simulink model "w1p2"  (R2020b)
settings: Solver=VariableStepAuto  StartTime=0.0  StopTime=100  MaxStep=0.0001  RelTol=1e-3
model workspace (MAT data in the model file):
  b = 20
  k1 = 50
  k2 = 200
  m1 = 150
  m2 = 100
settings Model: Creator=Puru Gawande  LastModifiedBy=family

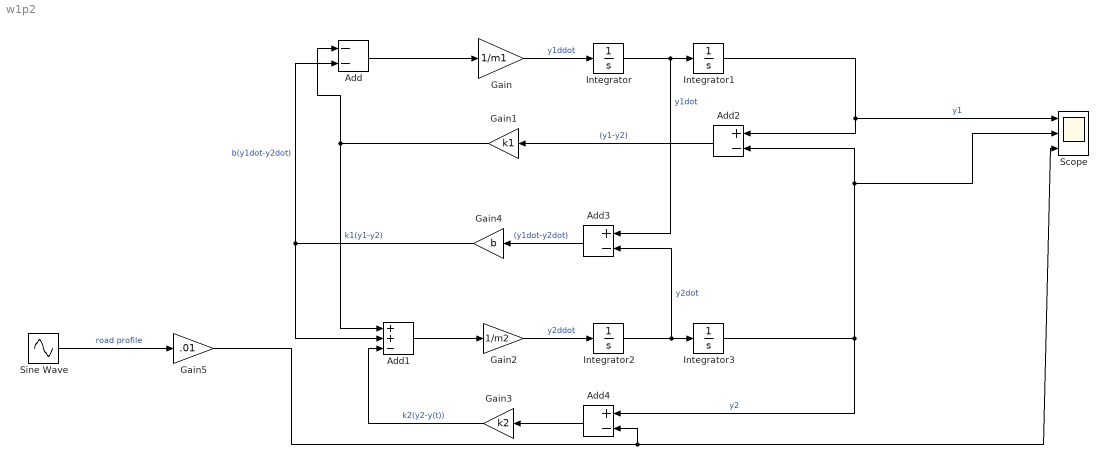
== system w1p2 ==
  Add : Sum  Inputs=--
  Add1 : Sum  Inputs=++-
  Add2 : Sum  Inputs=+-
  Add3 : Sum  Inputs=+-
  Add4 : Sum  Inputs=+-
  Gain : Gain  Gain=1/m1
  Gain1 : Gain  Gain=k1
  Gain2 : Gain  Gain=1/m2
  Gain3 : Gain  Gain=k2
  Gain4 : Gain  Gain=b
  Gain5 : Gain  Gain=.01
  Integrator{,1..3} (4 alike) : Integrator
  Scope : Scope  NumInputPorts=3
  Sine Wave : Sin  Amplitude=2  Frequency=10  SampleTime=0
  wires:
  Gain5/1 -> Add4/2, Scope/3
  Add4/1 -> Gain3/1
  Add2/1 -> Gain1/1  "(y1-y2)"
  Gain3/1 -> Add1/3  "k2(y2-y(t))"
  Gain/1 -> Integrator/1  "y1ddot"
  Add/1 -> Gain/1
  Gain2/1 -> Integrator2/1  "y2ddot"
  Integrator3/1 -> Add4/1, Scope/2, Add2/2  "y2"
  Integrator1/1 -> Add2/1, Scope/1  "y1"
  Gain4/1 -> Add1/2, Add/2  "b(y1dot-y2dot)"
  Sine Wave/1 -> Gain5/1  "road profile"
  Gain1/1 -> Add1/1, Add/1  "k1(y1-y2)"
  Integrator2/1 -> Add3/2, Integrator3/1  "y2dot"
  Add3/1 -> Gain4/1  "(y1dot-y2dot)"
  Integrator/1 -> Add3/1, Integrator1/1  "y1dot"
  Add1/1 -> Gain2/1
